simulink model "Comunicacion"  (R2021a)
settings: Solver=VariableStepAuto  StartTime=0.0  StopTime=inf  RelTol=1e-3
libraries: instrumentseriallib x2
settings Model: Creator=Avila  LastModifiedBy=Avila

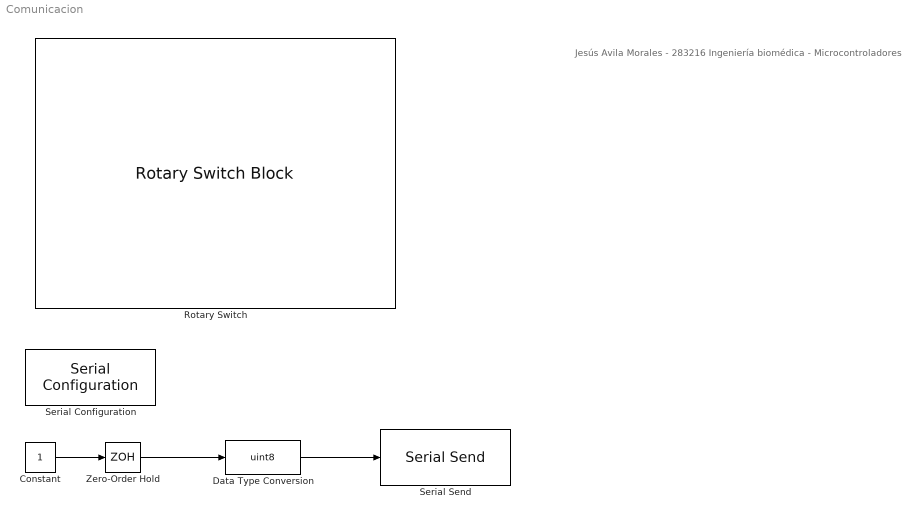
== system Comunicacion ==
  note: Jesús Avila Morales - 283216
      | Ingeniería biomédica - Microcontroladores
  Constant : Constant
  Data Type Conversion : DataTypeConversion  OutDataTypeStr=uint8
  Rotary Switch : RotarySwitchBlock
      settings: Values={{'0 %', '10 %', '20 %', '30 %', '40 %', '50 %', '60 %', '70 %', '80 %', '90 %', '100 %', 'Rojo', 'Verde', 'Azul'}, [1 10 20 30 40 50 60 70 80 90 100 114 118 97]}
  Serial Configuration : instrumentseriallib/Serial Configuration  Priority=-200000  Port=COM4  ComPort=COM4  BaudRate=9600  DataBits=8  Parity=none  StopBits=1  ByteOrder=little-endian  FlowControl=none  Timeout=10  SimulateUsing=Interpreted execution  BlockInModel=on
  Serial Send : instrumentseriallib/Serial Send  Priority=1  Port=COM4  ComPort=COM4  Header=[]  Terminator=<none>  CustomTerminator=[]  EnableBlockingMode=on  SimulateUsing=Interpreted execution  BlockInModel=on
  Zero-Order Hold : ZeroOrderHold  SampleTime=-1
  wires:
  Constant/1 -> Zero-Order Hold/1
  Zero-Order Hold/1 -> Data Type Conversion/1
  Data Type Conversion/1 -> Serial Send/1
